simulink model "ukupni_model_stari"  (Simulink 8.4)
settings: Solver=ode3  SolverMode=SingleTasking  StartTime=0.0  StopTime=inf  FixedStep=1e-3  RelTol=1e-3
values from neighbouring files (symbols this model uses):
  B_p = 0.08    [parametri.m]
  B_y = 0.14    [parametri.m]
  g = 9.81    [parametri.m]
  J_eq_y = J_y - m_heli*l_cm^2    (= 0.016488525)    [parametri.m]
  J_p = 0.0147    [parametri.m]
  K_i = lrq_i(A,B,Q,diag([3 3]))    [ise.m]
  K_pp = 0.25 * d_p    (= 0.04875)    [parametri.m]
  K_py = 0.01    [parametri.m]
  K_yp = 0.01    [parametri.m]
  K_yy = 0.25 * d_y    (= 0.04625)    [parametri.m]
  l_cm = 0.005    [parametri.m]
  m_heli = 2*(m_propeler + m_motor + m_motor_drzac) + m_sipka + m_drzac    (= 0.459)    [parametri.m]
undefined symbols (not defined in the file or in its folder): K_EC_P, K_EC_Y, max_u, MultiQ, PCI, Quanser, theta_0, Tr_p, Tr_y, wcf, zetaf
libraries: simulink_extras x5, rtwinlib x4, simulink x1
settings Model: Creator=Labos1  LastModifiedBy=Bojan  SimulationMode=external  CovMetricSettings=dwe  CovHtmlReporting=off  covSaveCumulativeToWorkspaceVar=off  CovSaveSingleToWorkspaceVar=off  CovExternalEMLEnable=on  CovSFcnEnable=on
settings SolverCC: PositivePriorityOrder=on
settings DataIOCC: LimitDataPoints=off  SaveFormat=StructureWithTime  SignalLoggingSaveFormat=Dataset
settings OptimizationCC: ExpressionDepthLimit=128
settings DebuggingCC: UnderspecifiedInitializationDetection=Simplified  MergeDetectMultiDrivingBlocksExec=error  SolverPrmCheckMsg=none  FcnCallInpInsideContextMsg=EnableAllAsError  FrameProcessingCompatibilityMsg=error  StateNameClashWarn=none  SFUnexpectedBacktrackingDiag=error  SFNoUnconditionalDefaultTransitionDiag=error
settings HardwareCC: ProdBitPerPointer=64  ProdLargestAtomicFloat=Float  ProdIntDivRoundTo=Zero  ProdEndianess=LittleEndian  ProdHWDeviceType=Specified
settings ModelReferenceCC: PropagateSignalLabelsOutOfModel=on
settings RTWCC: SystemTargetFile=rtwin.tlc  TemplateMakefile=rtwin.tmf  Description=Simulink Desktop Real-Time  RTWCompilerOptimization=On
settings CodeAppCC: MaxIdLength=95
settings RTWinTargetCC: TargetPreCompLibLocation=D:\Program Files\MATLAB\R2017a\toolbox\sldrt\lib\win64  TargetLangStandard=C99 (ISO)  GeneratePreprocessorConditionals=Use local settings  UseToolchainInfoCompliant=off  ExtModeMexFile=sldrtext

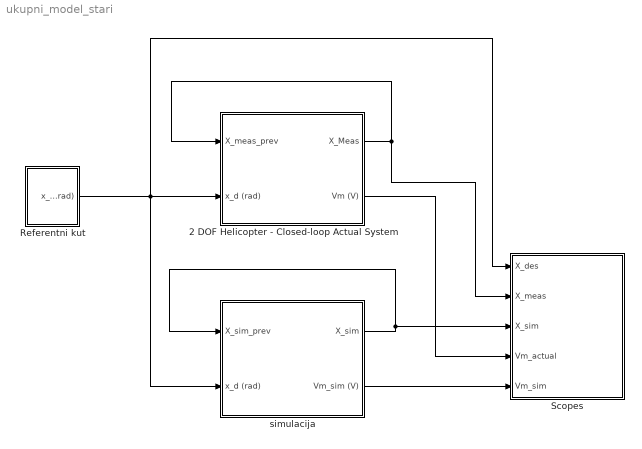
== system ukupni_model_stari ==
  2 DOF Helicopter - Closed-loop Actual System : Subsystem
  Referentni kut : Subsystem
  Scopes : Subsystem
  simulacija : Subsystem
  wires:
  simulacija/1(X_sim) -> simulacija/1(X_sim_prev), Scopes/3(X_sim)
  2 DOF Helicopter - Closed-loop Actual System/1(X_Meas) -> 2 DOF Helicopter - Closed-loop Actual System/1(X_meas_prev), Scopes/2(X_meas)
  2 DOF Helicopter - Closed-loop Actual System/2(Vm (V)) -> Scopes/4(Vm_actual)
  simulacija/2(Vm_sim (V)) -> Scopes/5(Vm_sim)
  Referentni kut/1(x_d (rad)) -> Scopes/1(X_des), 2 DOF Helicopter - Closed-loop Actual System/2(x_d (rad)), simulacija/2(x_d (rad))

== system ukupni_model_stari/2 DOF Helicopter - Closed-loop Actual System ==
  X_meas_prev : Inport
  x_d (rad) : Inport  Port=2
  2DOF HELI : Subsystem
  2DOF HELI: FF+LQR+I Controller : Subsystem
  X_Meas : Outport
  Vm (V) : Outport  Port=2
  wires:
  2DOF HELI/1(X_meas) -> X_Meas/1
  2DOF HELI/2(Vm (V)) -> Vm (V)/1
  x_d (rad)/1 -> 2DOF HELI: FF+LQR+I Controller/1(X_d (rad))
  X_meas_prev/1 -> 2DOF HELI: FF+LQR+I Controller/2(X)
  2DOF HELI: FF+LQR+I Controller/1(u_lqr_i_pitch (V)) -> 2DOF HELI/1(u_pitch (V))
  2DOF HELI: FF+LQR+I Controller/2(u_lqr_i_yaw (V)) -> 2DOF HELI/2(u_yaw (V))

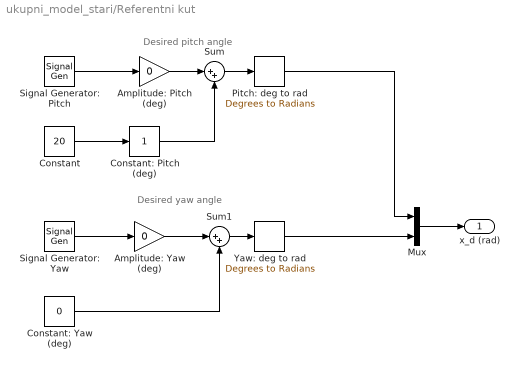
== system ukupni_model_stari/Referentni kut ==
  note: Desired pitch angle
  note: Desired yaw angle
  Amplitude: Pitch (deg) : Gain  Gain=0
  Amplitude: Yaw (deg) : Gain  Gain=0
  Constant : Constant  Value=20
  Constant: Pitch (deg) : simulink/Math Operations/Slider Gain  gain=1  low=1  high=2
  Constant: Yaw (deg) : Constant  Value=0
  Mux : Mux  Inputs=2
  Pitch: deg to rad : simulink_extras/Transformations/Degrees to Radians
  Signal Generator: Pitch : SignalGenerator  WaveForm=square  Amplitude=15  Frequency=0.05
  Signal Generator: Yaw : SignalGenerator  WaveForm=square  Amplitude=30  Frequency=0.05
  Sum : Sum  Inputs=|++
  Sum1 : Sum  Inputs=|++
  Yaw: deg to rad : simulink_extras/Transformations/Degrees to Radians
  x_d (rad) : Outport
  wires:
  Sum/1 -> Pitch: deg to rad/1
  Pitch: deg to rad/1 -> Mux/1
  Sum1/1 -> Yaw: deg to rad/1
  Amplitude: Yaw (deg)/1 -> Sum1/1
  Constant: Yaw (deg)/1 -> Sum1/2
  Mux/1 -> x_d (rad)/1
  Yaw: deg to rad/1 -> Mux/2
  Constant: Pitch (deg)/1 -> Sum/2
  Signal Generator: Yaw/1 -> Amplitude: Yaw (deg)/1
  Signal Generator: Pitch/1 -> Amplitude: Pitch (deg)/1
  Constant/1 -> Constant: Pitch (deg)/1
  Amplitude: Pitch (deg)/1 -> Sum/1

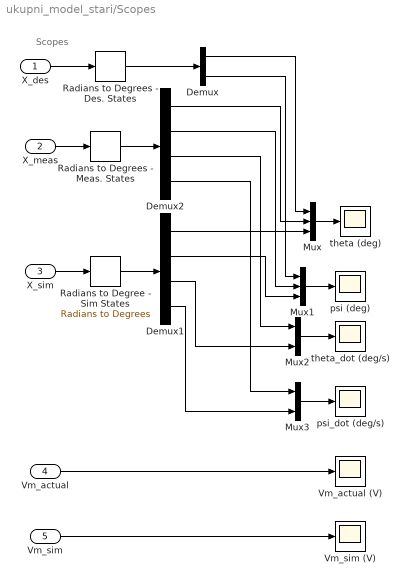
== system ukupni_model_stari/Scopes ==
  note: Scopes
  X_des : Inport
  X_meas : Inport  Port=2
  X_sim : Inport  Port=3
  Vm_actual : Inport  Port=4
  Vm_sim : Inport  Port=5
  Demux : Demux  Outputs=2
  Demux1 : Demux
  Demux2 : Demux
  Mux : Mux  Inputs=3
  Mux1 : Mux  Inputs=3
  Mux2 : Mux  Inputs=2
  Mux3 : Mux  Inputs=2
  Radians to Degree - Sim States : simulink_extras/Transformations/Radians to Degrees
  Radians to Degrees - Des. States : simulink_extras/Transformations/Radians to Degrees
  Radians to Degrees - Meas. States : simulink_extras/Transformations/Radians to Degrees
  Vm_actual (V) : Scope
      settings: TimeRange=auto  TickLabels=on  MaxDataPoints=5000  SaveName=Vm  YMin=-4.375  YMax=4.375  SampleTime=-1  DataFormat=Array
  Vm_sim (V) : Scope
      settings: TimeRange=1.000000  TickLabels=on  LimitDataPoints=on  MaxDataPoints=5000  SaveToWorkspace=off  SaveName=ScopeData5  YMin=-250  YMax=250  SampleTime=-1  DataFormat=Array
  psi (deg) : Scope
      settings: TimeRange=auto  TickLabels=on  MaxDataPoints=5000  SaveName=psi  YMin=-4.64301  YMax=11.84922  SampleTime=-1  DataFormat=Array
  psi_dot (deg/s) : Scope
      settings: TimeRange=1.000000  TickLabels=on  LimitDataPoints=on  MaxDataPoints=5000  SaveToWorkspace=off  SaveName=ScopeData3  YMin=-250  YMax=250  SampleTime=-1  DataFormat=Array
  theta (deg) : Scope
      settings: TimeRange=auto  TickLabels=on  MaxDataPoints=5000  SaveName=theta  YMin=19.9125  YMax=20.2875  SampleTime=-1  DataFormat=Array
  theta_dot (deg/s) : Scope
      settings: TimeRange=1.000000  TickLabels=on  LimitDataPoints=on  MaxDataPoints=5000  SaveToWorkspace=off  SaveName=ScopeData2  YMin=-250  YMax=250  SampleTime=-1  DataFormat=Array
  wires:
  Vm_sim/1 -> Vm_sim (V)/1
  Radians to Degrees - Des. States/1 -> Demux/1
  Demux1/2 -> Mux1/3
  Demux2/2 -> Mux1/2
  Demux/2 -> Mux1/1
  Demux1/1 -> Mux/3
  Demux2/1 -> Mux/2
  Demux/1 -> Mux/1
  X_des/1 -> Radians to Degrees - Des. States/1
  Demux2/3 -> Mux2/1
  Demux2/4 -> Mux3/1
  X_meas/1 -> Radians to Degrees - Meas. States/1
  Radians to Degrees - Meas. States/1 -> Demux2/1
  X_sim/1 -> Radians to Degree - Sim States/1
  Radians to Degree - Sim States/1 -> Demux1/1
  Mux/1 -> theta (deg)/1
  Mux1/1 -> psi (deg)/1
  Mux2/1 -> theta_dot (deg/s)/1
  Mux3/1 -> psi_dot (deg/s)/1
  Demux1/3 -> Mux2/2
  Demux1/4 -> Mux3/2
  Vm_actual/1 -> Vm_actual (V)/1

== system ukupni_model_stari/simulacija ==
  X_sim_prev : Inport
  x_d (rad) : Inport  Port=2
  kontroler : Subsystem
  model : Subsystem
  X_sim : Outport
  Vm_sim (V) : Outport  Port=2
  wires:
  x_d (rad)/1 -> kontroler/1(X_d (rad))
  X_sim_prev/1 -> kontroler/2(X)
  model/2(V_m_sim (V)) -> Vm_sim (V)/1
  model/1(X_sim) -> X_sim/1
  kontroler/1(u_lqr_i_pitch (V)) -> model/1(u_pitch (V))
  kontroler/2(u_lqr_i_yaw (V)) -> model/2(u_yaw (V))

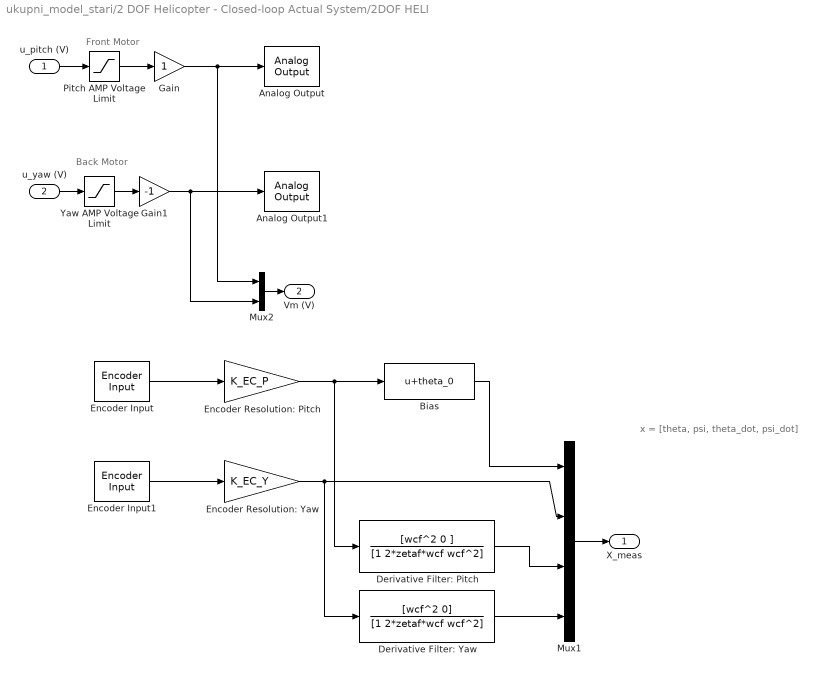
== system ukupni_model_stari/2 DOF Helicopter - Closed-loop Actual System/2DOF HELI ==
  note: Back Motor
  note: Front Motor
  note: x = [theta, psi, theta_dot, psi_dot]
  u_pitch (V) : Inport
  u_yaw (V) : Inport  Port=2
  Analog Output : rtwinlib/Analog Output  SampleTime=1e-3  MaxMissedTicks=10  ShowMissedTicks=off  YieldWhenWaiting=off  DrvName=Quanser/MultiQ-PCI  DrvAddress=4294967295  DrvOptions=zeros(1,0)  Channels=1  RangeMode=1  VoltRange=1  InitialValue=0  FinalValue=0
      settings: AttributesFormatString=Quanser\nMultiQ-PCI [auto]
  Analog Output1 : rtwinlib/Analog Output  SampleTime=1e-3  MaxMissedTicks=10  ShowMissedTicks=off  YieldWhenWaiting=off  DrvName=Quanser/MultiQ-PCI  DrvAddress=4294967295  DrvOptions=zeros(1,0)  Channels=2  RangeMode=1  VoltRange=1  InitialValue=0  FinalValue=0
      settings: AttributesFormatString=Quanser\nMultiQ-PCI [auto]
  Bias : Bias  Bias=theta_0
  Derivative Filter: Pitch : TransferFcn  Numerator=[wcf^2 0 ]  Denominator=[1 2*zetaf*wcf wcf^2]
  Derivative Filter: Yaw : TransferFcn  Numerator=[wcf^2 0]  Denominator=[1 2*zetaf*wcf wcf^2]
  Encoder Input : rtwinlib/Encoder Input  SampleTime=1e-3  MaxMissedTicks=10  ShowMissedTicks=off  YieldWhenWaiting=off  DrvName=Quanser/MultiQ-PCI  DrvAddress=4294967295  DrvOptions=zeros(1,0)  Channels=1  QuadMode=3  IndexPulse=2  InputFilter=Inf  DataType=1
      settings: AttributesFormatString=Quanser\nMultiQ-PCI [auto]
  Encoder Input1 : rtwinlib/Encoder Input  SampleTime=1e-3  MaxMissedTicks=10  ShowMissedTicks=off  YieldWhenWaiting=off  DrvName=Quanser/MultiQ-PCI  DrvAddress=4294967295  DrvOptions=zeros(1,0)  Channels=2  QuadMode=3  IndexPulse=2  InputFilter=Inf  DataType=1
      settings: AttributesFormatString=Quanser\nMultiQ-PCI [auto]
  "Encoder Resolution: Pitch " : Gain  Gain=K_EC_P
  Encoder Resolution: Yaw : Gain  Gain=K_EC_Y
  Gain : Gain
  Gain1 : Gain  Gain=-1
  Mux1 : Mux
  Mux2 : Mux  Inputs=2
  Pitch AMP Voltage Limit : Saturate  UpperLimit=max_u  LowerLimit=- max_u
  Yaw AMP Voltage Limit : Saturate  UpperLimit=max_u  LowerLimit=- max_u
  X_meas : Outport
  Vm (V) : Outport  Port=2
  wires:
  Encoder Resolution: Yaw/1 -> Mux1/2, Derivative Filter: Yaw/1
  Mux2/1 -> Vm (V)/1
  Mux1/1 -> X_meas/1
  u_yaw (V)/1 -> Yaw AMP Voltage Limit/1
  u_pitch (V)/1 -> Pitch AMP Voltage Limit/1
  Encoder Input/1 -> "Encoder Resolution: Pitch "/1
  "Encoder Resolution: Pitch "/1 -> Bias/1, Derivative Filter: Pitch/1
  Bias/1 -> Mux1/1
  Derivative Filter: Pitch/1 -> Mux1/3
  Derivative Filter: Yaw/1 -> Mux1/4
  Pitch AMP Voltage Limit/1 -> Gain/1
  Yaw AMP Voltage Limit/1 -> Gain1/1
  Encoder Input1/1 -> Encoder Resolution: Yaw/1
  Gain/1 -> Mux2/1, Analog Output/1
  Gain1/1 -> Analog Output1/1, Mux2/2

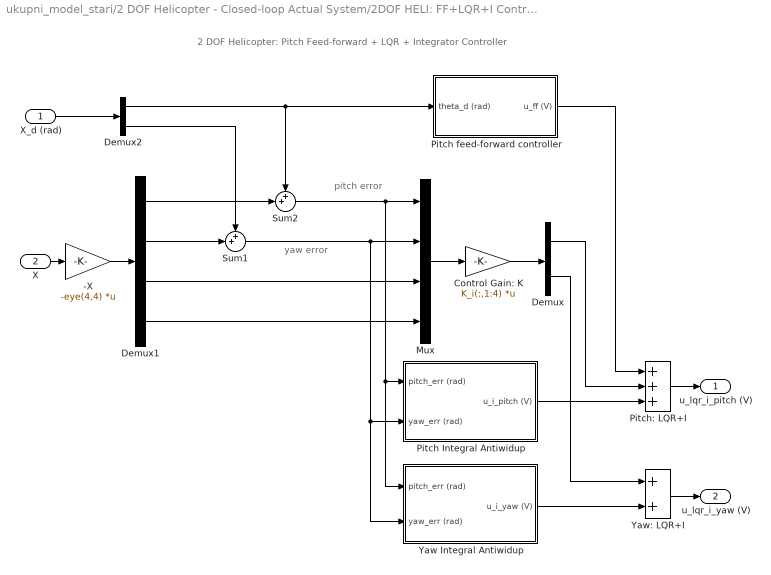
== system ukupni_model_stari/2 DOF Helicopter - Closed-loop Actual System/2DOF HELI: FF+LQR+I Controller ==
  note: yaw error
  note: pitch error
  note: 2 DOF Helicopter:
      | Pitch Feed-forward + LQR + Integrator Controller
  X_d (rad) : Inport
  X : Inport  Port=2
  -X : Gain  Gain=-eye(4,4)  Multiplication=Matrix(K*u)
  Control Gain: K : Gain  Gain=K_i(:,1:4)  Multiplication=Matrix(K*u)
  Demux : Demux  Outputs=2
  Demux1 : Demux
  Demux2 : Demux  Outputs=2
  Mux : Mux
  Pitch Integral Antiwidup : Subsystem
  Pitch feed-forward controller : Subsystem
  Pitch: LQR+I : Sum  Inputs=+++
  Sum1 : Sum  Inputs=++|
  Sum2 : Sum  Inputs=++|
  Yaw Integral Antiwidup : Subsystem
  Yaw: LQR+I : Sum
  u_lqr_i_pitch (V) : Outport
  u_lqr_i_yaw (V) : Outport  Port=2
  wires:
  Demux1/2 -> Sum1/2
  Demux2/2 -> Sum1/1
  Demux2/1 -> Sum2/1, Pitch feed-forward controller/1(theta_d (rad))
  X_d (rad)/1 -> Demux2/1
  Yaw Integral Antiwidup/1(u_i_yaw (V)) -> Yaw: LQR+I/2
  Demux/2 -> Yaw: LQR+I/1
  Yaw: LQR+I/1 -> u_lqr_i_yaw (V)/1
  Pitch: LQR+I/1 -> u_lqr_i_pitch (V)/1
  Demux/1 -> Pitch: LQR+I/2
  Pitch Integral Antiwidup/1(u_i_pitch (V)) -> Pitch: LQR+I/3
  Pitch feed-forward controller/1(u_ff (V)) -> Pitch: LQR+I/1
  Sum2/1 -> Mux/1, Yaw Integral Antiwidup/1(pitch_err (rad)), Pitch Integral Antiwidup/1(pitch_err (rad))
  Demux1/1 -> Sum2/2
  X/1 -> -X/1
  Sum1/1 -> Yaw Integral Antiwidup/2(yaw_err (rad)), Pitch Integral Antiwidup/2(yaw_err (rad)), Mux/2
  -X/1 -> Demux1/1
  Control Gain: K/1 -> Demux/1
  Mux/1 -> Control Gain: K/1
  Demux1/3 -> Mux/3
  Demux1/4 -> Mux/4

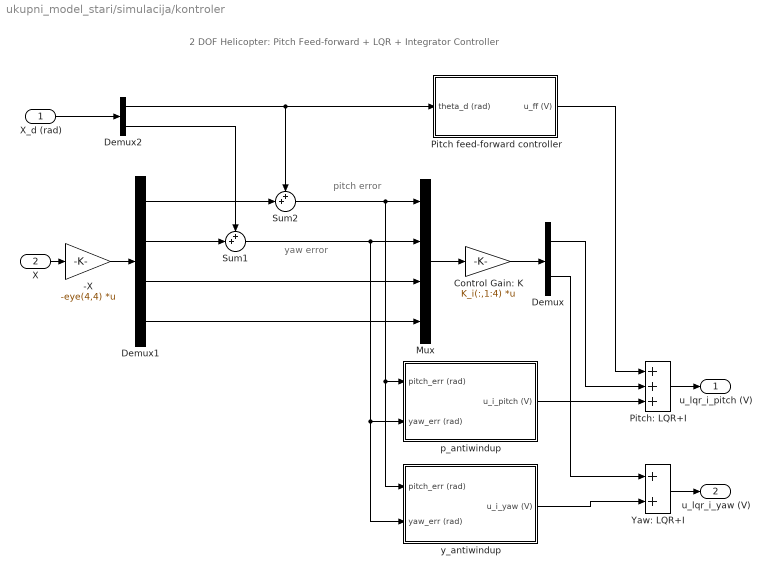
== system ukupni_model_stari/simulacija/kontroler ==
  note: yaw error
  note: pitch error
  note: 2 DOF Helicopter:
      | Pitch Feed-forward + LQR + Integrator Controller
  X_d (rad) : Inport
  X : Inport  Port=2
  -X : Gain  Gain=-eye(4,4)  Multiplication=Matrix(K*u)
  Control Gain: K : Gain  Gain=K_i(:,1:4)  Multiplication=Matrix(K*u)
  Demux : Demux  Outputs=2
  Demux1 : Demux
  Demux2 : Demux  Outputs=2
  Mux : Mux
  Pitch feed-forward controller : Subsystem
  Pitch: LQR+I : Sum  Inputs=+++
  Sum1 : Sum  Inputs=++|
  Sum2 : Sum  Inputs=++|
  Yaw: LQR+I : Sum
  p_antiwindup : Subsystem
  y_antiwindup : Subsystem
  u_lqr_i_pitch (V) : Outport
  u_lqr_i_yaw (V) : Outport  Port=2
  wires:
  Demux1/2 -> Sum1/2
  Demux2/2 -> Sum1/1
  Demux2/1 -> Sum2/1, Pitch feed-forward controller/1(theta_d (rad))
  X_d (rad)/1 -> Demux2/1
  y_antiwindup/1(u_i_yaw (V)) -> Yaw: LQR+I/2
  Demux/2 -> Yaw: LQR+I/1
  Yaw: LQR+I/1 -> u_lqr_i_yaw (V)/1
  Pitch: LQR+I/1 -> u_lqr_i_pitch (V)/1
  Demux/1 -> Pitch: LQR+I/2
  p_antiwindup/1(u_i_pitch (V)) -> Pitch: LQR+I/3
  Pitch feed-forward controller/1(u_ff (V)) -> Pitch: LQR+I/1
  Sum2/1 -> Mux/1, y_antiwindup/1(pitch_err (rad)), p_antiwindup/1(pitch_err (rad))
  Demux1/1 -> Sum2/2
  X/1 -> -X/1
  Sum1/1 -> y_antiwindup/2(yaw_err (rad)), p_antiwindup/2(yaw_err (rad)), Mux/2
  -X/1 -> Demux1/1
  Control Gain: K/1 -> Demux/1
  Mux/1 -> Control Gain: K/1
  Demux1/3 -> Mux/3
  Demux1/4 -> Mux/4

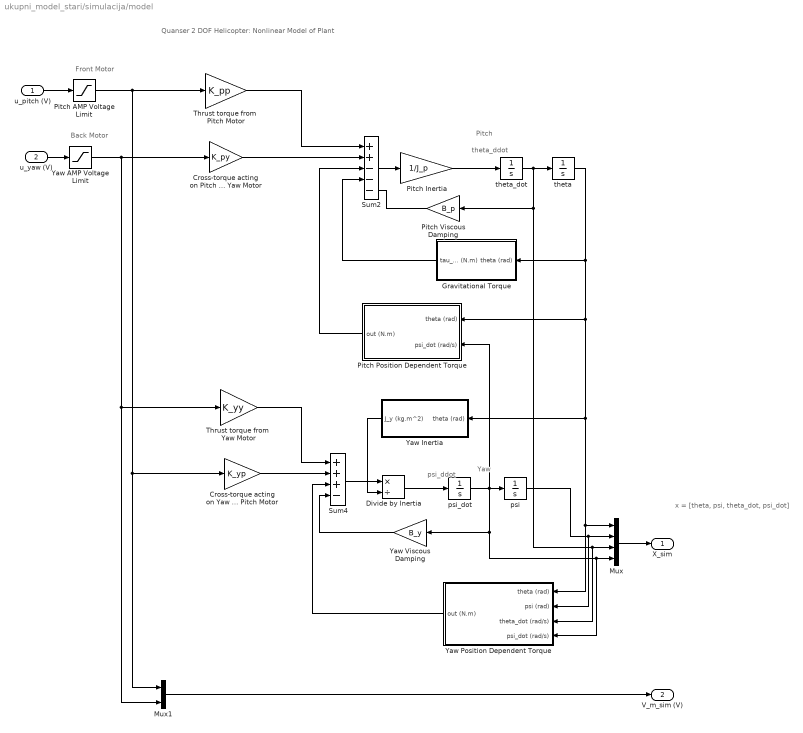
== system ukupni_model_stari/simulacija/model ==
  note: Back Motor
  note: Front Motor
  note: x = [theta, psi, theta_dot, psi_dot]
  note: Quanser 2 DOF Helicopter: Nonlinear Model of Plant
  note: theta_ddot
  note: psi_ddot
  note: Pitch
  note: Yaw
  u_pitch (V) : Inport
  u_yaw (V) : Inport  Port=2
  Cross-torque acting on Pitch  from Yaw Motor : Gain  Gain=K_py
  Cross-torque acting on Yaw  from Pitch Motor : Gain  Gain=K_yp
  Divide by Inertia : Product  Inputs=*/
  Gravitational Torque : Subsystem
  Mux : Mux
  Mux1 : Mux  Inputs=2
  Pitch AMP Voltage Limit : Saturate  UpperLimit=max_u  LowerLimit=- max_u
  Pitch Inertia : Gain  Gain=1/J_p
  Pitch Position Dependent Torque : Subsystem
  Pitch Viscous Damping : Gain  Gain=B_p
  Sum2 : Sum  Inputs=++---
  Sum4 : Sum  Inputs=+++-
  Thrust torque from  Pitch Motor : Gain  Gain=K_pp
  Thrust torque from  Yaw Motor : Gain  Gain=K_yy
  Yaw AMP Voltage Limit : Saturate  UpperLimit=max_u  LowerLimit=- max_u
  Yaw Inertia : Subsystem
  Yaw Position Dependent Torque : Subsystem
  Yaw Viscous Damping : Gain  Gain=B_y
  psi : Integrator
  psi_dot : Integrator
  theta : Integrator  InitialCondition=theta_0  LimitOutput=on  UpperSaturationLimit=60*pi/180  LowerSaturationLimit=-60*pi/180
  theta_dot : Integrator
  X_sim : Outport
  V_m_sim (V) : Outport  Port=2
  wires:
  Pitch Position Dependent Torque/1(out (N.m)) -> Sum2/3
  Gravitational Torque/1(tau_g (N.m)) -> Sum2/4
  Pitch Viscous Damping/1 -> Sum2/5
  Cross-torque acting on Pitch  from Yaw Motor/1 -> Sum2/2
  Thrust torque from  Pitch Motor/1 -> Sum2/1
  Yaw Inertia/1(J_y (kg.m^2)) -> Divide by Inertia/2
  Divide by Inertia/1 -> psi_dot/1
  Sum4/1 -> Divide by Inertia/1
  Yaw Position Dependent Torque/1(out (N.m)) -> Sum4/3
  Yaw Viscous Damping/1 -> Sum4/4
  psi/1 -> Yaw Position Dependent Torque/2(psi (rad)), Mux/2
  Mux1/1 -> V_m_sim (V)/1
  Yaw AMP Voltage Limit/1 -> Thrust torque from  Yaw Motor/1, Mux1/2, Cross-torque acting on Pitch  from Yaw Motor/1
  Pitch AMP Voltage Limit/1 -> Mux1/1, Cross-torque acting on Yaw  from Pitch Motor/1, Thrust torque from  Pitch Motor/1
  Mux/1 -> X_sim/1
  theta/1 -> Gravitational Torque/1(theta (rad)), Pitch Position Dependent Torque/1(theta (rad)), Yaw Position Dependent Torque/1(theta (rad)), Mux/1, Yaw Inertia/1(theta (rad))
  Sum2/1 -> Pitch Inertia/1
  Pitch Inertia/1 -> theta_dot/1
  theta_dot/1 -> Pitch Viscous Damping/1, Yaw Position Dependent Torque/3(theta_dot (rad/s)), Mux/3, theta/1
  Thrust torque from  Yaw Motor/1 -> Sum4/1
  Cross-torque acting on Yaw  from Pitch Motor/1 -> Sum4/2
  psi_dot/1 -> Yaw Viscous Damping/1, Yaw Position Dependent Torque/4(psi_dot (rad/s)), Mux/4, Pitch Position Dependent Torque/2(psi_dot (rad/s)), psi/1
  u_pitch (V)/1 -> Pitch AMP Voltage Limit/1
  u_yaw (V)/1 -> Yaw AMP Voltage Limit/1

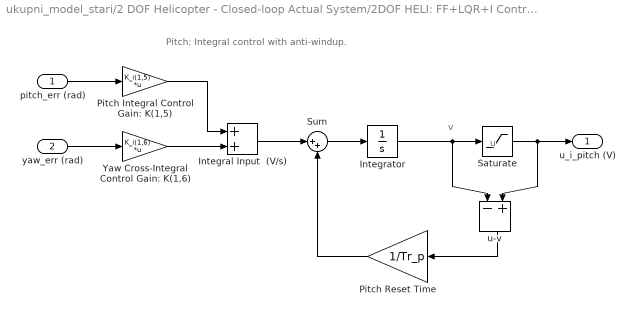
== system ukupni_model_stari/2 DOF Helicopter - Closed-loop Actual System/2DOF HELI: FF+LQR+I Controller/Pitch Integral Antiwidup ==
  note: Pitch: Integral control with anti-windup.
  note: v
  note: u
  pitch_err (rad) : Inport
  yaw_err (rad) : Inport  Port=2
  Integral Input  (V/s) : Sum
  Integrator : Integrator
  Pitch Integral Control Gain: K(1,5) : Gain  Gain=K_i(1,5)  Multiplication=Matrix(K*u)
  Pitch Reset Time : Gain  Gain=1/Tr_p
  Saturate : Saturate  UpperLimit=max_u  LowerLimit=-max_u
  Sum : Sum  Inputs=|++
  Yaw Cross-Integral Control Gain: K(1,6) : Gain  Gain=K_i(1,6)  Multiplication=Matrix(K*u)
  u-v : Sum  Inputs=-+
  u_i_pitch (V) : Outport
  wires:
  Integral Input  (V/s)/1 -> Sum/1
  Yaw Cross-Integral Control Gain: K(1,6)/1 -> Integral Input  (V/s)/2
  Pitch Integral Control Gain: K(1,5)/1 -> Integral Input  (V/s)/1
  yaw_err (rad)/1 -> Yaw Cross-Integral Control Gain: K(1,6)/1
  Pitch Reset Time/1 -> Sum/2
  Sum/1 -> Integrator/1
  u-v/1 -> Pitch Reset Time/1
  Saturate/1 -> u-v/2, u_i_pitch (V)/1
  Integrator/1 -> Saturate/1, u-v/1
  pitch_err (rad)/1 -> Pitch Integral Control Gain: K(1,5)/1

== system ukupni_model_stari/2 DOF Helicopter - Closed-loop Actual System/2DOF HELI: FF+LQR+I Controller/Pitch feed-forward controller ==
  note: Desired pitch angle
  theta_d (rad) : Inport
  Feed-forward Pitch Gain : Gain  Gain=l_cm*m_heli*g / K_pp
  Trigonometric Function : Trigonometry  Operator=cos  OutputSignalType=real
  u_ff (V) : Outport
  wires:
  theta_d (rad)/1 -> Trigonometric Function/1
  Feed-forward Pitch Gain/1 -> u_ff (V)/1
  Trigonometric Function/1 -> Feed-forward Pitch Gain/1

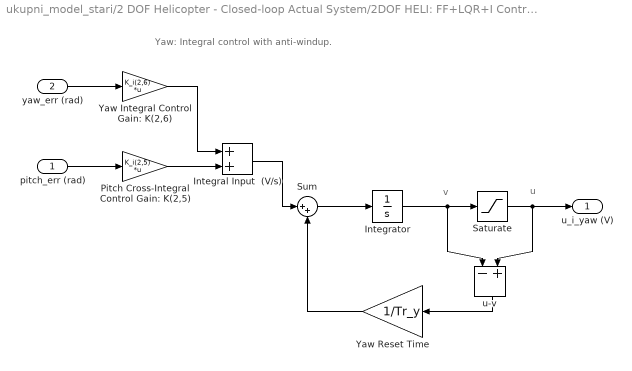
== system ukupni_model_stari/2 DOF Helicopter - Closed-loop Actual System/2DOF HELI: FF+LQR+I Controller/Yaw Integral Antiwidup ==
  note: Yaw: Integral control with anti-windup.
  note: u
  note: v
  pitch_err (rad) : Inport
  yaw_err (rad) : Inport  Port=2
  Integral Input  (V/s) : Sum
  Integrator : Integrator
  Pitch Cross-Integral Control Gain: K(2,5) : Gain  Gain=K_i(2,5)  Multiplication=Matrix(K*u)
  Saturate : Saturate  UpperLimit=max_u  LowerLimit=-max_u
  Sum : Sum  Inputs=|++
  Yaw Integral Control Gain: K(2,6) : Gain  Gain=K_i(2,6)  Multiplication=Matrix(K*u)
  Yaw Reset Time : Gain  Gain=1/Tr_y
  u-v : Sum  Inputs=-+
  u_i_yaw (V) : Outport
  wires:
  Integral Input  (V/s)/1 -> Sum/1
  Pitch Cross-Integral Control Gain: K(2,5)/1 -> Integral Input  (V/s)/2
  Yaw Integral Control Gain: K(2,6)/1 -> Integral Input  (V/s)/1
  pitch_err (rad)/1 -> Pitch Cross-Integral Control Gain: K(2,5)/1
  yaw_err (rad)/1 -> Yaw Integral Control Gain: K(2,6)/1
  Integrator/1 -> u-v/1, Saturate/1
  Saturate/1 -> u_i_yaw (V)/1, u-v/2
  u-v/1 -> Yaw Reset Time/1
  Sum/1 -> Integrator/1
  Yaw Reset Time/1 -> Sum/2

== system ukupni_model_stari/simulacija/kontroler/Pitch feed-forward controller ==
  note: Desired pitch angle
  theta_d (rad) : Inport
  Feed-forward Pitch Gain : Gain  Gain=l_cm*m_heli*g / K_pp
  Trigonometric Function : Trigonometry  Operator=cos  OutputSignalType=real
  u_ff (V) : Outport
  wires:
  theta_d (rad)/1 -> Trigonometric Function/1
  Feed-forward Pitch Gain/1 -> u_ff (V)/1
  Trigonometric Function/1 -> Feed-forward Pitch Gain/1

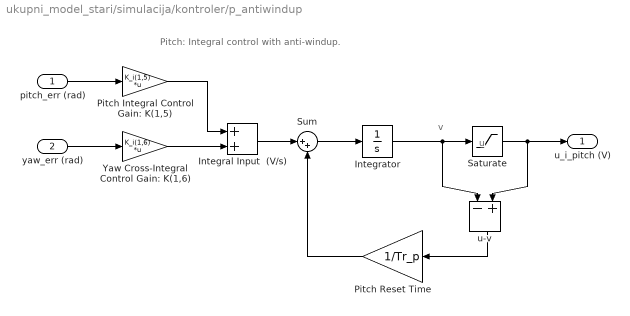
== system ukupni_model_stari/simulacija/kontroler/p_antiwindup ==
  note: Pitch: Integral control with anti-windup.
  note: v
  note: u
  pitch_err (rad) : Inport
  yaw_err (rad) : Inport  Port=2
  Integral Input  (V/s) : Sum
  Integrator : Integrator
  Pitch Integral Control Gain: K(1,5) : Gain  Gain=K_i(1,5)  Multiplication=Matrix(K*u)
  Pitch Reset Time : Gain  Gain=1/Tr_p
  Saturate : Saturate  UpperLimit=max_u  LowerLimit=-max_u
  Sum : Sum  Inputs=|++
  Yaw Cross-Integral Control Gain: K(1,6) : Gain  Gain=K_i(1,6)  Multiplication=Matrix(K*u)
  u-v : Sum  Inputs=-+
  u_i_pitch (V) : Outport
  wires:
  Integral Input  (V/s)/1 -> Sum/1
  Yaw Cross-Integral Control Gain: K(1,6)/1 -> Integral Input  (V/s)/2
  Pitch Integral Control Gain: K(1,5)/1 -> Integral Input  (V/s)/1
  yaw_err (rad)/1 -> Yaw Cross-Integral Control Gain: K(1,6)/1
  Pitch Reset Time/1 -> Sum/2
  Sum/1 -> Integrator/1
  u-v/1 -> Pitch Reset Time/1
  Saturate/1 -> u-v/2, u_i_pitch (V)/1
  Integrator/1 -> Saturate/1, u-v/1
  pitch_err (rad)/1 -> Pitch Integral Control Gain: K(1,5)/1

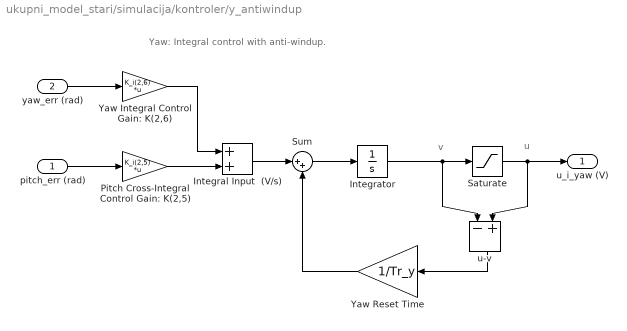
== system ukupni_model_stari/simulacija/kontroler/y_antiwindup ==
  note: Yaw: Integral control with anti-windup.
  note: u
  note: v
  pitch_err (rad) : Inport
  yaw_err (rad) : Inport  Port=2
  Integral Input  (V/s) : Sum
  Integrator : Integrator
  Pitch Cross-Integral Control Gain: K(2,5) : Gain  Gain=K_i(2,5)  Multiplication=Matrix(K*u)
  Saturate : Saturate  UpperLimit=max_u  LowerLimit=-max_u
  Sum : Sum  Inputs=|++
  Yaw Integral Control Gain: K(2,6) : Gain  Gain=K_i(2,6)  Multiplication=Matrix(K*u)
  Yaw Reset Time : Gain  Gain=1/Tr_y
  u-v : Sum  Inputs=-+
  u_i_yaw (V) : Outport
  wires:
  Integral Input  (V/s)/1 -> Sum/1
  Pitch Cross-Integral Control Gain: K(2,5)/1 -> Integral Input  (V/s)/2
  Yaw Integral Control Gain: K(2,6)/1 -> Integral Input  (V/s)/1
  pitch_err (rad)/1 -> Pitch Cross-Integral Control Gain: K(2,5)/1
  yaw_err (rad)/1 -> Yaw Integral Control Gain: K(2,6)/1
  Integrator/1 -> u-v/1, Saturate/1
  Saturate/1 -> u_i_yaw (V)/1, u-v/2
  u-v/1 -> Yaw Reset Time/1
  Sum/1 -> Integrator/1
  Yaw Reset Time/1 -> Sum/2

== system ukupni_model_stari/simulacija/model/Gravitational Torque ==
  theta (rad) : Inport
  Trigonometric Function : Trigonometry  Operator=cos  OutputSignalType=real
  m*g*lcm : Gain  Gain=m_heli*g*l_cm
  tau_g (N.m) : Outport
  wires:
  m*g*lcm/1 -> tau_g (N.m)/1
  theta (rad)/1 -> Trigonometric Function/1
  Trigonometric Function/1 -> m*g*lcm/1

== system ukupni_model_stari/simulacija/model/Pitch Position Dependent Torque ==
  theta (rad) : Inport
  psi_dot (rad/s) : Inport  Port=2
  Product : Product  Inputs=4  RndMeth=Zero
  cos(theta) : Trigonometry  Operator=cos  OutputSignalType=real
  m*lcm^2 : Gain  Gain=m_heli*l_cm^2
  sin(theta) : Trigonometry  OutputSignalType=real
  out (N.m) : Outport
  wires:
  psi_dot (rad/s)/1 -> Product/4, Product/3
  theta (rad)/1 -> cos(theta)/1, sin(theta)/1
  Product/1 -> m*lcm^2/1
  sin(theta)/1 -> Product/1
  cos(theta)/1 -> Product/2
  m*lcm^2/1 -> out (N.m)/1

== system ukupni_model_stari/simulacija/model/Yaw Inertia ==
  theta (rad) : Inport
  Sum3 : Sum
  Yaw Inertia : Constant  Value=J_eq_y
  cos(theta) : Trigonometry  Operator=cos  OutputSignalType=real
  cos(theta)^2 : Product  RndMeth=Zero
  m_heli*l_cm^2 : Gain  Gain=m_heli*l_cm^2
  J_y (kg.m^2) : Outport
  wires:
  cos(theta)/1 -> cos(theta)^2/2, cos(theta)^2/1
  Sum3/1 -> J_y (kg.m^2)/1
  theta (rad)/1 -> cos(theta)/1
  m_heli*l_cm^2/1 -> Sum3/2
  Yaw Inertia/1 -> Sum3/1
  cos(theta)^2/1 -> m_heli*l_cm^2/1

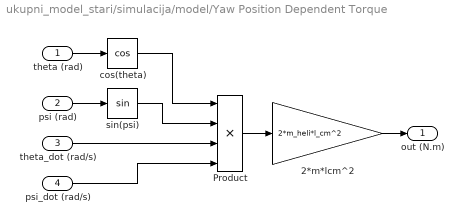
== system ukupni_model_stari/simulacija/model/Yaw Position Dependent Torque ==
  theta (rad) : Inport
  psi (rad) : Inport  Port=2
  theta_dot (rad/s) : Inport  Port=3
  psi_dot (rad/s) : Inport  Port=4
  2*m*lcm^2 : Gain  Gain=2*m_heli*l_cm^2
  Product : Product  Inputs=4  RndMeth=Zero
  cos(theta) : Trigonometry  Operator=cos  OutputSignalType=real
  sin(psi) : Trigonometry  OutputSignalType=real
  out (N.m) : Outport
  wires:
  2*m*lcm^2/1 -> out (N.m)/1
  psi_dot (rad/s)/1 -> Product/4
  theta_dot (rad/s)/1 -> Product/3
  sin(psi)/1 -> Product/2
  cos(theta)/1 -> Product/1
  Product/1 -> 2*m*lcm^2/1
  theta (rad)/1 -> cos(theta)/1
  psi (rad)/1 -> sin(psi)/1
